simulink model "SimulinkschaltbildTeil3"  (R2014b)
settings: Solver=ode45  StartTime=0.0  StopTime=10.0  RelTol=1e-3
settings Model: Creator=Florian  LastModifiedBy=Florian

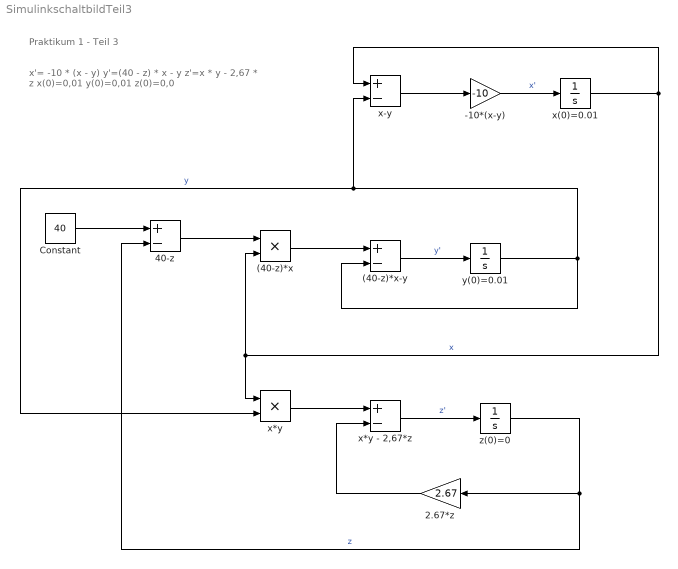
== system SimulinkschaltbildTeil3 ==
  note: Praktikum 1 - Teil 3
  note: x'= -10 * (x - y)
      | y'=(40 - z) * x - y
      | z'=x * y - 2,67 * z
      |
      | x(0)=0,01 y(0)=0,01 z(0)=0,0
  (40-z)*x : Product
  (40-z)*x-y : Sum  Inputs=+-
  -10*(x-y) : Gain  Gain=-10
  2.67*z : Gain  Gain=2.67
  40-z : Sum  Inputs=+-
  Constant : Constant  Value=40
  x(0)=0.01 : Integrator
  x*y : Product
  x*y - 2,67*z : Sum  Inputs=+-
  x-y : Sum  Inputs=+-
  y(0)=0.01 : Integrator
  z(0)=0 : Integrator
  wires:
  x(0)=0.01/1 -> x*y/1, (40-z)*x/2, x-y/1  "x"
  (40-z)*x-y/1 -> y(0)=0.01/1  "y'"
  y(0)=0.01/1 -> (40-z)*x-y/2, x*y/2, x-y/2  "y"
  Constant/1 -> 40-z/1
  40-z/1 -> (40-z)*x/1
  (40-z)*x/1 -> (40-z)*x-y/1
  x-y/1 -> -10*(x-y)/1
  -10*(x-y)/1 -> x(0)=0.01/1  "x'"
  x*y/1 -> x*y - 2,67*z/1
  x*y - 2,67*z/1 -> z(0)=0/1  "z'"
  z(0)=0/1 -> 2.67*z/1, 40-z/2  "z"
  2.67*z/1 -> x*y - 2,67*z/2
